simulink model "spacecraft_attitude_model"  (R2024b)
settings: Solver=ode4  StartTime=t0  StopTime=tf  FixedStep=0.1  RelTol=1e-3
values from neighbouring files (symbols this model uses):
  a = (((T/(2*pi))^2*mu_earth)^(1/3))    (= 7069867.85099)    [main_spacecraft_attitude_dynamics.m]
  A_body1 = surface(1)    [main_spacecraft_attitude_dynamics.m]
  A_body2 = surface(2)    [main_spacecraft_attitude_dynamics.m]
  A_body3 = surface(3)    [main_spacecraft_attitude_dynamics.m]
  A_body4 = surface(4)    [main_spacecraft_attitude_dynamics.m]
  A_body5 = surface(5)    [main_spacecraft_attitude_dynamics.m]
  A_body6 = surface(6)    [main_spacecraft_attitude_dynamics.m]
  A_panel1 = surface(7)    [main_spacecraft_attitude_dynamics.m]
  A_panel2 = surface(8)    [main_spacecraft_attitude_dynamics.m]
  A_panel3 = surface(9)    [main_spacecraft_attitude_dynamics.m]
  A_panel4 = surface(10)    [main_spacecraft_attitude_dynamics.m]
  alpha = [alpha1,alpha2,alpha3]    [main_spacecraft_attitude_dynamics.m]
  Ap = pinv(Ar)    [main_spacecraft_attitude_dynamics.m]
  Ar = Ar./norm(Ar)    [main_spacecraft_attitude_dynamics.m]
  AtmosphereModel = struct()    [AtmosphereData.m]    (also in main_spacecraft_attitude_dynamics.m)
  CD = 2.6    [main_spacecraft_attitude_dynamics.m]
  D_max = 50    [main_spacecraft_attitude_dynamics.m]
  Detumbling_time = 5000    [main_spacecraft_attitude_dynamics.m]
  e = 0.001    [main_spacecraft_attitude_dynamics.m]
  FOV = 128 * pi/180    (= 2.23402144255)    [main_spacecraft_attitude_dynamics.m]
  g1_0 = DGRF2020(1).g_nm    [main_spacecraft_attitude_dynamics.m]
  g1_1 = DGRF2020(2).g_nm    [main_spacecraft_attitude_dynamics.m]
  H = 700    [main_spacecraft_attitude_dynamics.m]
  h0 = 0    [main_spacecraft_attitude_dynamics.m]
  h1_1 = DGRF2020(2).h_nm    [main_spacecraft_attitude_dynamics.m]
  i = deg2rad(98.18)    [main_spacecraft_attitude_dynamics.m]
  Ir = 0.1    [main_spacecraft_attitude_dynamics.m]
  J = EXTRACTED_DATA.I_total    [main_spacecraft_attitude_dynamics.m]
  j_B = [0.01, 0.05, 0.01]'    [main_spacecraft_attitude_dynamics.m]
  k1 = max(max(kd_slew))    [main_spacecraft_attitude_dynamics.m]
  k2 = max(max(kp_slew))    [main_spacecraft_attitude_dynamics.m]
  Kw = max(max(kp_detumbling))    [main_spacecraft_attitude_dynamics.m]
  n = sqrt((G*M_E)/(r_earth^3))    [main_spacecraft_attitude_dynamics.m]
  N_B1 = N_B(1, :)'    [main_spacecraft_attitude_dynamics.m]
  N_B2 = N_B(2, :)'    [main_spacecraft_attitude_dynamics.m]
  N_B3 = N_B(3, :)'    [main_spacecraft_attitude_dynamics.m]
  N_B4 = N_B(4, :)'    [main_spacecraft_attitude_dynamics.m]
  N_B5 = N_B(5, :)'    [main_spacecraft_attitude_dynamics.m]
  N_B6 = N_B(6, :)'    [main_spacecraft_attitude_dynamics.m]
  N_P1 = N_B(7, :)'    [main_spacecraft_attitude_dynamics.m]
  N_P2 = N_B(8, :)'    [main_spacecraft_attitude_dynamics.m]
  N_P3 = N_B(9, :)'    [main_spacecraft_attitude_dynamics.m]
  N_P4 = N_B(10, :)'    [main_spacecraft_attitude_dynamics.m]
  n_S = (2*pi)/T_S    (= 1.99238499086e-07)    [main_spacecraft_attitude_dynamics.m]
  om = deg2rad(0)    [main_spacecraft_attitude_dynamics.m]
  P = Fe/c    (= 4.52980041279e-06)    [main_spacecraft_attitude_dynamics.m]
  pd_body1 = rho_D(1)    [main_spacecraft_attitude_dynamics.m]
  pd_body2 = rho_D(2)    [main_spacecraft_attitude_dynamics.m]
  pd_body3 = rho_D(3)    [main_spacecraft_attitude_dynamics.m]
  pd_body4 = rho_D(4)    [main_spacecraft_attitude_dynamics.m]
  pd_body5 = rho_D(5)    [main_spacecraft_attitude_dynamics.m]
  pd_body6 = rho_D(6)    [main_spacecraft_attitude_dynamics.m]
  pd_panel1 = rho_D(7)    [main_spacecraft_attitude_dynamics.m]
  pd_panel2 = rho_D(8)    [main_spacecraft_attitude_dynamics.m]
  pd_panel3 = rho_D(9)    [main_spacecraft_attitude_dynamics.m]
  pd_panel4 = rho_D(10)    [main_spacecraft_attitude_dynamics.m]
  ps_body1 = rho_S(1)    [main_spacecraft_attitude_dynamics.m]
  ps_body2 = rho_S(2)    [main_spacecraft_attitude_dynamics.m]
  ps_body3 = rho_S(3)    [main_spacecraft_attitude_dynamics.m]
  ps_body4 = rho_S(4)    [main_spacecraft_attitude_dynamics.m]
  ps_body5 = rho_S(5)    [main_spacecraft_attitude_dynamics.m]
  ps_body6 = rho_S(6)    [main_spacecraft_attitude_dynamics.m]
  ps_panel1 = rho_S(7)    [main_spacecraft_attitude_dynamics.m]
  ps_panel2 = rho_S(8)    [main_spacecraft_attitude_dynamics.m]
  ps_panel3 = rho_S(9)    [main_spacecraft_attitude_dynamics.m]
  ps_panel4 = rho_S(10)    [main_spacecraft_attitude_dynamics.m]
  q0 = [q1_0 q2_0 q3_0 q4_0]    [main_spacecraft_attitude_dynamics.m]
  r_earth = (R_earth + H)*10^3    (= 7078136.3)    [main_spacecraft_attitude_dynamics.m]
  R_earth = 6378.1363    [main_spacecraft_attitude_dynamics.m]
  r_f1 = r_F(1, :)'    [main_spacecraft_attitude_dynamics.m]
  r_f10 = r_F(10, :)'    [main_spacecraft_attitude_dynamics.m]
  r_f2 = r_F(2, :)'    [main_spacecraft_attitude_dynamics.m]
  r_f3 = r_F(3, :)'    [main_spacecraft_attitude_dynamics.m]
  r_f4 = r_F(4, :)'    [main_spacecraft_attitude_dynamics.m]
  r_f5 = r_F(5, :)'    [main_spacecraft_attitude_dynamics.m]
  r_f6 = r_F(6, :)'    [main_spacecraft_attitude_dynamics.m]
  r_f7 = r_F(7, :)'    [main_spacecraft_attitude_dynamics.m]
  r_f8 = r_F(8, :)'    [main_spacecraft_attitude_dynamics.m]
  r_f9 = r_F(9, :)'    [main_spacecraft_attitude_dynamics.m]
  r_Sun = 149597870    [main_spacecraft_attitude_dynamics.m]
  RAAN = deg2rad(RAAN)    [main_spacecraft_attitude_dynamics.m]
  sigma_b = RRW*(pi/180)*(1/3600)*(1/sqrt(Ts))    [main_spacecraft_attitude_dynamics.m]
  sigma_mag = 10^-6    (= 1e-06)    [main_spacecraft_attitude_dynamics.m]
  sigma_n = ARW*(pi/180)*(1/60)*(1/sqrt(Ts))    [main_spacecraft_attitude_dynamics.m]
  T_coil_max = 50 * 45*10^-6    (= 0.00225)    [main_spacecraft_attitude_dynamics.m]
  th0 = 0    [main_spacecraft_attitude_dynamics.m]
  v0 = [0 0 0]    [main_spacecraft_attitude_dynamics.m]
  variance_Ss = (a_sun)^2    (= 3.24)    [main_spacecraft_attitude_dynamics.m]
  w_0 = [-3, 3, 3]'    [main_spacecraft_attitude_dynamics.m]
  w_E = (2*pi)/(24*60*60)    (= 7.27220521664e-05)    [main_spacecraft_attitude_dynamics.m]
  w_LN = [0 0 0]'    [main_spacecraft_attitude_dynamics.m]
undefined symbols (not defined in the file or in its folder): A_Ss_orienation
libraries: matrix_library x38, slpidlib x2, aerolibutil x1, vrlib x1
(part 1 of 4)
settings Model: Creator=pmarzai02  LastModifiedBy=paolo
settings DebuggingCC: AlgebraicLoopMsg=none

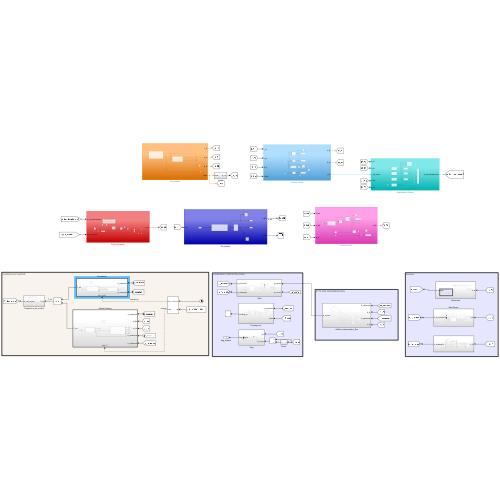
[thumbnail: Simulink's stored preview of the top-level diagram]
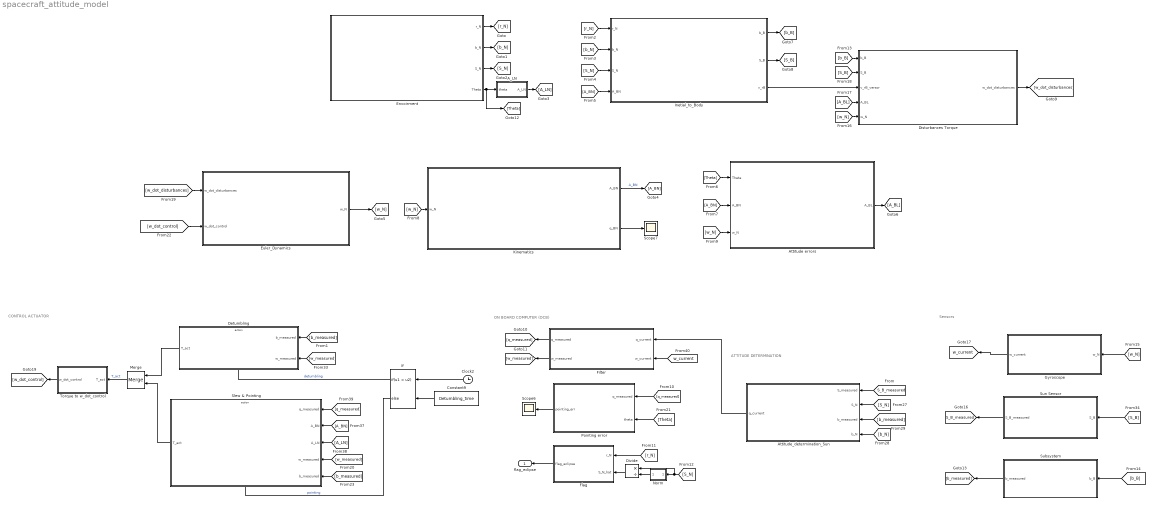
== system spacecraft_attitude_model ==
  note: CONTROL ACTUATOR
  note: ON BOARD COMPUTER (OCB)
  note: Sensors
  note: ATTITUDE DETERMINATION
  " Filter" : Subsystem
  A_LN : Subsystem
  Attitude errors : Subsystem
  Attitude_determination_Sun : Subsystem
  Clock2 : Clock
  Constant9 : Constant  Value=Detumbling_time
  Detumbling : Subsystem  TreatAsAtomicUnit=on
  Disturbances Torque : Subsystem
  Divide : Product  Inputs=*/
  Envoirment : Subsystem
  Euler_Dynamics : Subsystem
  Flag : Subsystem
  Gyroscope : Subsystem
  If : If  NumInputs=2  IfExpression=u1 < u2
  Inetial_to_Body : Subsystem
  Kinematics : Subsystem
  Merge : Merge
  Norm : Subsystem
  Pointing error : Subsystem
  Scope6 : Scope
  Scope7 : Scope
  Slew & Pointing : Subsystem  TreatAsAtomicUnit=on
  Subsystem : Subsystem
  "Sun Sensor " : Subsystem
  Torque to w_dot_control : Subsystem
  flag_eclipse : Outport
  tag scope: S_B_measured=global, w_current=global
  wires:
  Envoirment/1(r_N) -> [r_N]
  Envoirment/2(b_N) -> [b_N]
  Envoirment/3(S_N) -> [S_N]
  [r_N] -> Inetial_to_Body/1(r_N)
  [b_N] -> Inetial_to_Body/2(b_N)
  [S_N] -> Inetial_to_Body/3(S_N)
  Kinematics/1(A_BN) -> [A_BN]  "A_BN"
  [A_BN] -> Inetial_to_Body/4(A_BN)
  [Theta] -> Attitude errors/1(Theta)
  [A_BN] -> Attitude errors/2(A_BN)
  Euler_Dynamics/1(w_N) -> [w_N]
  [w_N] -> Kinematics/1(w_N)
  [w_N] -> Attitude errors/3(w_N)
  [w_N] -> Disturbances Torque/5(w_N)
  [A_BL] -> Disturbances Torque/4(A_BL)
  Attitude errors/1(A_BL) -> [A_BL]
  Inetial_to_Body/1(b_B) -> [b_B]
  Inetial_to_Body/2(S_B) -> [S_B]
  [b_B] -> Disturbances Torque/1(b_B)
  [S_B] -> Disturbances Torque/2(S_B)
  Disturbances Torque/1(w_dot_disturbances) -> [w_dot_disturbances]
  [w_dot_disturbances] -> Euler_Dynamics/1(w_dot_disturbances)
  Subsystem/1(b_measured) -> [b_measured]
  Kinematics/2(q_BN) -> Scope7/1
  Inetial_to_Body/3(v_rB) -> Disturbances Torque/3(v_rB_versor)
  Divide/1 -> Flag/2(S_N_hat)
  [r_N] -> Flag/1(r_N)
  Norm/1(Out1) -> Divide/2
  Flag/1(flag_eclipse) -> flag_eclipse/1
  "Sun Sensor "/1(S_B_measured) -> [S_B_measured]
  [S_B] -> "Sun Sensor "/1(S_B)
  Envoirment/4(Theta) -> [Theta], A_LN/1(theta)
  [b_measured] -> Attitude_determination_Sun/3(b_measured)
  [S_N] -> Attitude_determination_Sun/2(S_N)
  [S_B_measured] -> Attitude_determination_Sun/1(S_measured)
  [b_N] -> Attitude_determination_Sun/4(b_N)
  [w_current] -> " Filter"/2(w_current)
  A_LN/1("A_LN ") -> [A_LN]
  [w_N] -> Gyroscope/1(w_N)
  Gyroscope/1(w_current) -> [w_current]
  [b_B] -> Subsystem/1(b_B)
  [S_N] -> Divide/1, Norm/1(In1)
  " Filter"/1(q_measured) -> [q_measured]
  " Filter"/2(w_measured) -> [w_measured]
  Attitude_determination_Sun/1(q_current) -> " Filter"/1(q_current)
  Constant9/1 -> If/2
  Clock2/1 -> If/1
  If/1 -> Detumbling/Action  "detumbling"
  Detumbling/1(T_act) -> Merge/1
  [b_measured] -> Detumbling/1(b_measured)
  [w_measured] -> Detumbling/2(w_measured)
  [q_measured] -> Pointing error/1(q_measured)
  [Theta] -> Pointing error/2(theta)
  Pointing error/1(pointing_err) -> Scope6/1
  Merge/1 -> Torque to w_dot_control/1(T_act)  "T_act"
  Torque to w_dot_control/1("w_dot_control ") -> [w_dot_control]
  [w_dot_control] -> Euler_Dynamics/2("w_dot_control ")
  If/2 -> Slew & Pointing/Action  "pointing"
  [w_measured] -> Slew & Pointing/4(w_measured)
  [q_measured] -> Slew & Pointing/1(q_measured)
  [A_BN] -> Slew & Pointing/2(A_BN)
  [A_LN] -> Slew & Pointing/3(A_LN)
  [b_measured] -> Slew & Pointing/5(b_measured)
  Slew & Pointing/1(T_act) -> Merge/2

== system spacecraft_attitude_model/ Filter ==
  note: try different Ki and Kp
  q_current : Inport
  w_current : Inport  Port=2
  Clock : Clock
  PID Controller : slpidlib/PID Controller  Controller=PID  Form=Parallel  TimeDomain=Continuous-time  UseExternalTs=off  SampleTime=-1  IntegratorMethod=Forward Euler  FilterMethod=Forward Euler  ControllerParametersSource=internal  P=0.00001  I=0.00000001  UseKiTs=off  D=0  UseExternalDerivativeSource=off  N=100  UseFilter=on  TunerSelectOption=Transfer Function Based (PID Tuner App)  InitialConditionSource=internal  InitialConditionForIntegrator=0  InitialConditionForFilter=0  DifferentiatorICPrevScaledInput=0  ExternalReset=none  TrackingMode=off  Kt=1  LimitOutput=off  SatLimitsSource=internal  UpperSaturationLimit=inf  LowerSaturationLimit=-inf  LinearizeAsGain=on  AntiWindupMode=none  Kb=1  LimitIntegrator=off  UpperIntegratorSaturationLimit=inf  LowerIntegratorSaturationLimit=-inf  POutMin=[]  POutMax=[]  IOutMin=[]  IOutMax=[]  DOutMin=[]  DOutMax=[]  NOutMin=[]  NOutMax=[]  SumOutMin=[]  SumOutMax=[]  SaturationOutMin=[]  SaturationOutMax=[]  PParamMin=[]  PParamMax=[]  IParamMin=[]  IParamMax=[]  DParamMin=[]  DParamMax=[]  NParamMin=[]  NParamMax=[]  KbParamMin=[]  KbParamMax=[]  KtParamMin=[]  KtParamMax=[]  KbOutMin=[]  KbOutMax=[]  KtOutMin=[]  KtOutMax=[]  IntegratorOutMin=[]  IntegratorOutMax=[]  FilterOutMin=[]  FilterOutMax=[]  SumI1OutMin=[]  SumI1OutMax=[]  SumI2OutMin=[]  SumI2OutMax=[]  SumI3OutMin=[]  SumI3OutMax=[]  SumI4OutMin=[]  SumI4OutMax=[]  SumDOutMin=[]  SumDOutMax=[]  DifferentiatorOutMin=[]  DifferentiatorOutMax=[]  FilterDiffOutCoefMin=[]  FilterDiffOutCoefMax=[]  ReciprocalOutMin=[]  ReciprocalOutMax=[]  SumDenOutMin=[]  SumDenOutMax=[]  SumNumOutMin=[]  SumNumOutMax=[]  DivideOutMin=[]  DivideOutMax=[]  UdiffTsProdOutMin=[]  UdiffTsProdOutMax=[]  NTsProdOutMin=[]  NTsProdOutMax=[]  UintegralTsProdOutMin=[]  UintegralTsProdOutMax=[]  UngainTsProdOutMin=[]  UngainTsProdOutMax=[]  ClampingZeroOutDataTypeStr=Inherit: Inherit via back propagation  ClampingZeroOutMin=[]  ClampingZeroOutMax=[]  FilterDenConstantOutDataTypeStr=Inherit: Inherit via back propagation  FilterDenConstantOutMin=[]  FilterDenConstantOutMax=[]  PCopyOutDataTypeStr=Inherit: Inherit via back propagation  PCopyOutMin=[]  PCopyOutMax=[]  NCopyOutDataTypeStr=Inherit: Inherit via back propagation  NCopyOutMin=[]  NCopyOutMax=[]  IntegratorContinuousStateAttributes=''  IntegratorStateMustResolveToSignalObject=off  IntegratorRTWStateStorageClass=Auto  FilterContinuousStateAttributes=''  FilterStateMustResolveToSignalObject=off  FilterRTWStateStorageClass=Auto  ParallelPVariant=InternalParameters  IdealPVariant=Disabled  IVariant=InternalParameters  DVariant=InternalParameters  IntegratorVariant=Continuous  SatVariant=Disabled  AWVariant=Passthrough  PCopyVariant=Disabled  TRVariant=Disabled  FdbkBlocksVariant=Forward  IdealPFdbkVariant=Disabled  SatFdbkVariant=Disabled  DerivativeFilterVariant=ContFilter  NVariant=InternalParameters  NCopyVariant=Disabled  FilterICVariant=InternalICsFilter  IntegratorICVariant=InternalICs  ExternalResetVariant=Disabled  TRSumVariant=Passthrough  SumFdbkVariant=Disabled  SumVariant=Sum_PID  TsampFilterVariant=InternalTs  TsampNgainVariant=Passthrough  TsampIntegralVariant=Disabled_SignalSpec  ExternalSaturationOutDataTypeStr=Inherit: Same as second input  DerivativeSourceVariant=ErrorSignal  PreIntVariant=InternalPreInt
  Quaternions : Subsystem
  Scope : Scope
  Scope2 : Scope
  Scope5 : Scope
  Selector : Selector  InputPortWidth=4  IndexOptions=Index vector (dialog)  Indices=[1:3]  OutputSizes=1
  Subsystem : Subsystem
  Sum : Sum  Inputs=++|
  Switch : Switch  Criteria=u2 > Threshold  SaturateOnIntegerOverflow=off  InputSameDT=off
  To Workspace : ToWorkspace  VariableName=q_measured  SampleTime=-1
  To Workspace1 : ToWorkspace  VariableName=w_measured  SampleTime=-1
  Zero-Order Hold1 : ZeroOrderHold  SampleTime=0.1
  q_measured : Outport
  w_measured : Outport  Port=2
  wires:
  Subsystem/1(q_error) -> Selector/1
  PID Controller/1 -> Scope5/1, Sum/2
  w_current/1 -> Sum/1
  Selector/1 -> PID Controller/1
  Clock/1 -> Switch/2
  Quaternions/1(quaternions) -> Switch/1, Zero-Order Hold1/1
  Switch/1 -> Subsystem/2(q_measured)
  q_current/1 -> Switch/3, Subsystem/1(q_referance)
  Sum/1 -> Quaternions/1(w_current), To Workspace1/1, Scope/1, w_measured/1
  Zero-Order Hold1/1 -> Scope2/1, To Workspace/1, q_measured/1

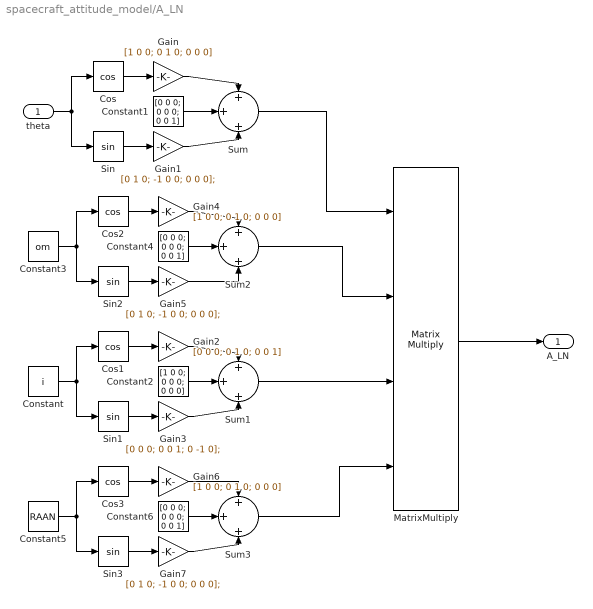
== system spacecraft_attitude_model/A_LN ==
  theta : Inport
  Constant : Constant  Value=i
  Constant1 : Constant  Value=[0 0 0; 0 0 0; 0 0 1]
  Constant2 : Constant  Value=[1 0 0; 0 0 0; 0 0 0]
  Constant3 : Constant  Value=om
  Constant4 : Constant  Value=[0 0 0; 0 0 0; 0 0 1]
  Constant5 : Constant  Value=RAAN
  Constant6 : Constant  Value=[0 0 0; 0 0 0; 0 0 1]
  Cos{,1..3} (4 alike) : Trigonometry  Operator=cos
  Gain : Gain  Gain=[1 0 0; 0 1 0; 0 0 0]
  Gain1 : Gain  Gain=[0 1 0; -1 0 0; 0 0 0];
  Gain2 : Gain  Gain=[0 0 0; 0 1 0; 0 0 1]
  Gain3 : Gain  Gain=[0 0 0; 0 0 1; 0 -1 0];
  Gain4 : Gain  Gain=[1 0 0; 0 1 0; 0 0 0]
  Gain5 : Gain  Gain=[0 1 0; -1 0 0; 0 0 0];
  Gain6 : Gain  Gain=[1 0 0; 0 1 0; 0 0 0]
  Gain7 : Gain  Gain=[0 1 0; -1 0 0; 0 0 0];
  MatrixMultiply : Product  Inputs=4  Multiplication=Matrix(*)
  Sin{,1..3} (4 alike) : Trigonometry
  Sum{,1..3} (4 alike) : Sum  Inputs=+||+||+
  "A_LN " : Outport
  wires:
  theta/1 -> Sin/1, Cos/1
  Cos/1 -> Gain/1
  Sin/1 -> Gain1/1
  Gain1/1 -> Sum/3
  Gain/1 -> Sum/1
  Constant1/1 -> Sum/2
  Sum/1 -> MatrixMultiply/1
  Constant/1 -> Sin1/1, Cos1/1
  Constant2/1 -> Sum1/2
  Sin1/1 -> Gain3/1
  Gain3/1 -> Sum1/3
  Cos1/1 -> Gain2/1
  Sum1/1 -> MatrixMultiply/3
  Gain2/1 -> Sum1/1
  MatrixMultiply/1 -> "A_LN "/1
  Sum2/1 -> MatrixMultiply/2
  Gain4/1 -> Sum2/1
  Cos2/1 -> Gain4/1
  Constant3/1 -> Sin2/1, Cos2/1
  Constant4/1 -> Sum2/2
  Gain5/1 -> Sum2/3
  Sin2/1 -> Gain5/1
  Sum3/1 -> MatrixMultiply/4
  Gain6/1 -> Sum3/1
  Cos3/1 -> Gain6/1
  Constant5/1 -> Sin3/1, Cos3/1
  Constant6/1 -> Sum3/2
  Gain7/1 -> Sum3/3
  Sin3/1 -> Gain7/1

== system spacecraft_attitude_model/Attitude errors ==
  Theta : Inport
  A_BN : Inport  Port=2
  w_N : Inport  Port=3
  A_LN : Subsystem
  Constant : Constant  Value=w_LN
  Gain : Gain  Gain=-1
  Matrix Multiply : Product  Multiplication=Matrix(*)
  Matrix Multiply1 : Product  Multiplication=Matrix(*)
  Scope : Scope
  Scope1 : Scope
  Sum : Sum  Inputs=|++
  To Workspace : ToWorkspace  VariableName=A_BL  SampleTime=-1
  To Workspace1 : ToWorkspace  VariableName=w_BL  SampleTime=-1
  Transpose : matrix_library/Transpose
  A_BL : Outport
  wires:
  A_BN/1 -> Matrix Multiply/1
  Matrix Multiply/1 -> Matrix Multiply1/1, A_BL/1, To Workspace/1, Scope1/1
  Matrix Multiply1/1 -> Gain/1
  Gain/1 -> Sum/2
  w_N/1 -> Sum/1
  Sum/1 -> Scope/1, To Workspace1/1
  A_LN/1(A_LN) -> Transpose/1
  Transpose/1 -> Matrix Multiply/2
  Constant/1 -> Matrix Multiply1/2
  Theta/1 -> A_LN/1(Theta)

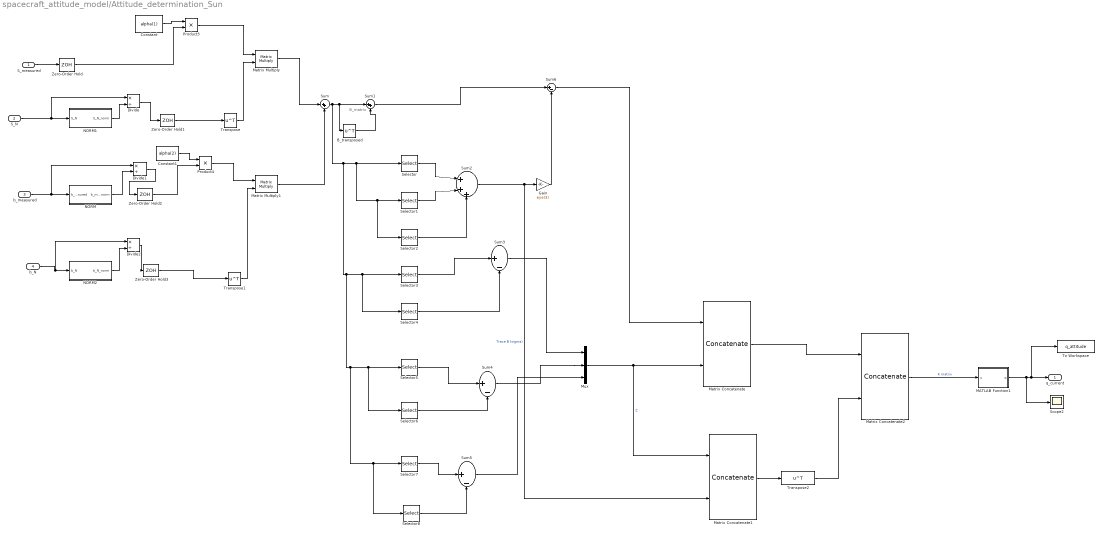
== system spacecraft_attitude_model/Attitude_determination_Sun ==
  note: B_matrix
  S_measured : Inport
  S_N : Inport  Port=2
  b_measured : Inport  Port=3
  b_N : Inport  Port=4
  B_transposed : Math  Operator=transpose
  Constant : Constant  Value=alpha(1)
  Constant1 : Constant  Value=alpha(2)
  Divide : Product  Inputs=*/
  Divide1 : Product  Inputs=*/
  Divide2 : Product  Inputs=*/
  Gain : Gain  Gain=eye(3)
  MATLAB Function1 : MATLAB Function  TreatAsAtomicUnit=on
  Matrix Concatenate : Concatenate  Mode=Multidimensional array  ConcatenateDimension=2
  Matrix Concatenate1 : Concatenate  Mode=Multidimensional array
  Matrix Concatenate2 : Concatenate  Mode=Multidimensional array
  Matrix Multiply : Product  Multiplication=Matrix(*)
  Matrix Multiply1 : Product  Multiplication=Matrix(*)
  Mux : Mux  Inputs=3
  NORM : Subsystem
  NORM1 : Subsystem
  NORM2 : Subsystem
  Product3 : Product
  Product4 : Product
  Scope2 : Scope
  Selector : Selector  NumberOfDimensions=2  InputPortWidth=3  IndexOptions=Index vector (dialog),Index vector (dialog)  Indices=[1],1  OutputSizes=1,1
  Selector1 : Selector  NumberOfDimensions=2  InputPortWidth=3  IndexOptions=Index vector (dialog),Index vector (dialog)  Indices=[2],2  OutputSizes=1,1
  Selector2 : Selector  NumberOfDimensions=2  InputPortWidth=3  IndexOptions=Index vector (dialog),Index vector (dialog)  Indices=[3],3  OutputSizes=1,1
  Selector3 : Selector  NumberOfDimensions=2  InputPortWidth=3  IndexOptions=Index vector (dialog),Index vector (dialog)  Indices=[2],3  OutputSizes=1,1
  Selector4 : Selector  NumberOfDimensions=2  InputPortWidth=3  IndexOptions=Index vector (dialog),Index vector (dialog)  Indices=[3],2  OutputSizes=1,1
  Selector5 : Selector  NumberOfDimensions=2  InputPortWidth=3  IndexOptions=Index vector (dialog),Index vector (dialog)  Indices=[3],1  OutputSizes=1,1
  Selector6 : Selector  NumberOfDimensions=2  InputPortWidth=3  IndexOptions=Index vector (dialog),Index vector (dialog)  Indices=[1],3  OutputSizes=1,1
  Selector7 : Selector  NumberOfDimensions=2  InputPortWidth=3  IndexOptions=Index vector (dialog),Index vector (dialog)  Indices=[1],2  OutputSizes=1,1
  Selector8 : Selector  NumberOfDimensions=2  InputPortWidth=3  IndexOptions=Index vector (dialog),Index vector (dialog)  Indices=[2],1  OutputSizes=1,1
  Sum : Sum  Inputs=|++
  Sum1 : Sum  Inputs=|++
  Sum2 : Sum  Inputs=|+++
  Sum{3..6} (4 alike) : Sum  Inputs=|+-
  To Workspace : ToWorkspace  VariableName=q_attitude  SampleTime=-1
  Transpose : Math  Operator=transpose
  Transpose1 : Math  Operator=transpose
  Transpose2 : Math  Operator=transpose
  Zero-Order Hold{,1..3} (4 alike) : ZeroOrderHold  SampleTime=-1
  q_current : Outport
  wires:
  b_measured/1 -> Divide1/1, NORM/1(b_measured)
  S_N/1 -> Divide/1, NORM1/1(S_N)
  b_N/1 -> Divide2/1, NORM2/1(b_N)
  S_measured/1 -> Zero-Order Hold/1
  Zero-Order Hold/1 -> Product3/2
  Zero-Order Hold1/1 -> Transpose/1
  Zero-Order Hold2/1 -> Product4/2
  Zero-Order Hold3/1 -> Transpose1/1
  NORM1/1(S_N_norm) -> Divide/2
  Divide/1 -> Zero-Order Hold1/1
  NORM/1(b_measured_norm) -> Divide1/2
  Divide1/1 -> Zero-Order Hold2/1
  NORM2/1(b_N_norm) -> Divide2/2
  Divide2/1 -> Zero-Order Hold3/1
  Constant/1 -> Product3/1
  Transpose/1 -> Matrix Multiply/2
  Product3/1 -> Matrix Multiply/1
  Matrix Multiply/1 -> Sum/1
  Constant1/1 -> Product4/1
  Product4/1 -> Matrix Multiply1/1
  Transpose1/1 -> Matrix Multiply1/2
  Matrix Multiply1/1 -> Sum/2
  Sum/1 -> Selector8/1, Selector7/1, Selector6/1, Selector5/1, Selector4/1, Selector3/1, Selector2/1, Selector1/1, Selector/1, Sum1/1, B_transposed/1
  B_transposed/1 -> Sum1/2
  Selector/1 -> Sum2/1
  Selector1/1 -> Sum2/2
  Selector2/1 -> Sum2/3
  Sum2/1 -> Matrix Concatenate1/2, Gain/1  "Trace B (sigma)"
  Selector3/1 -> Sum3/1
  Selector4/1 -> Sum3/2
  Selector5/1 -> Sum4/1
  Selector6/1 -> Sum4/2
  Selector7/1 -> Sum5/1
  Selector8/1 -> Sum5/2
  Sum3/1 -> Mux/1
  Sum4/1 -> Mux/2
  Sum5/1 -> Mux/3
  Mux/1 -> Matrix Concatenate1/1, Matrix Concatenate/2  "Z"
  Sum1/1 -> Sum6/1
  Gain/1 -> Sum6/2
  Sum6/1 -> Matrix Concatenate/1
  Matrix Concatenate1/1 -> Transpose2/1
  Matrix Concatenate/1 -> Matrix Concatenate2/1
  Transpose2/1 -> Matrix Concatenate2/2
  Matrix Concatenate2/1 -> MATLAB Function1/1(u)  "K matrix"
  MATLAB Function1/1(q) -> Scope2/1, To Workspace/1, q_current/1

== system spacecraft_attitude_model/Detumbling ==
  b_measured : Inport
  w_measured : Inport  Port=2
  Action Port : ActionPort  ActionPortLabel=if(u1 < u2)
  Detumbling : Subsystem
  Subsystem4 : Subsystem
  T_act : Outport
  wires:
  b_measured/1 -> Subsystem4/2(b_measured)
  Detumbling/1(T_detumbling) -> Subsystem4/1(T_control)
  w_measured/1 -> Subsystem4/3(w_measured), Detumbling/1(w_measured)
  Subsystem4/1(T_act) -> T_act/1

== system spacecraft_attitude_model/Disturbances Torque ==
  b_B : Inport
  S_B : Inport  Port=2
  v_rB_versor : Inport  Port=3
  A_BL : Inport  Port=4
  w_N : Inport  Port=5
  Air Drag : Subsystem
  Gain{,1..3} (4 alike) : Gain
  Gravity Gradient : Subsystem
  Magnetic_Torque : Subsystem
  Scope : Scope  NumInputPorts=4
  Solar_Radiation_Torque : Subsystem
  Sum : Sum  Inputs=|++++
  torque to w_dot_B : Subsystem
  torque to w_dot_Drag : Subsystem
  torque to w_dot_SRP : Subsystem
  w_dot_disturbances : Outport
  wires:
  Solar_Radiation_Torque/1(T sun) -> Scope/2, torque to w_dot_SRP/1(T_S)  "T_SRP"
  Gravity Gradient/1(w_dot_GG) -> Gain3/1
  Gain1/1 -> Sum/2
  w_N/1 -> Gravity Gradient/2(w)
  b_B/1 -> Magnetic_Torque/1(b_B)
  Gain2/1 -> Sum/3
  Gain3/1 -> Sum/4
  Air Drag/1(T_Drag) -> Scope/3, torque to w_dot_Drag/1(T_Drag)  "T_DRAG"
  torque to w_dot_SRP/1("w_dot_SRP ") -> Gain/1
  torque to w_dot_B/1(w_dot_B) -> Gain1/1
  Gain/1 -> Sum/1
  torque to w_dot_Drag/1(w_dot_Drag) -> Gain2/1
  v_rB_versor/1 -> Air Drag/1(v_rB_versor)
  A_BL/1 -> Gravity Gradient/1(A_BL)
  S_B/1 -> Solar_Radiation_Torque/1(S_B)
  Sum/1 -> w_dot_disturbances/1
  Gravity Gradient/2("T_GG ") -> Scope/4  "T_GG"
  Magnetic_Torque/1(T_B) -> Scope/1, torque to w_dot_B/1(T_B)  "T_M"

== system spacecraft_attitude_model/Envoirment ==
  Model : Subsystem
  Scope : Scope
  Two_Body_Keplerian_Dynamics : Subsystem
  r_N : Outport
  b_N : Outport  Port=2
  S_N : Outport  Port=3
  Theta : Outport  Port=4
  wires:
  Two_Body_Keplerian_Dynamics/1(r_N) -> r_N/1, Model/1(r_N)
  Model/1(b_N) -> Scope/1, b_N/1
  Model/2(S_N) -> S_N/1
  Two_Body_Keplerian_Dynamics/2(Theta) -> Theta/1

== system spacecraft_attitude_model/Euler_Dynamics ==
  note: Euler's equation in vectorial forme
      | $I*\underline{\dot{\omega}} + \underline{{\omega}} \times (I * \underline{{\omega}}) = T$
      | It has needed a vector of initial angular speed $\omega_0$
      | $\underline{\dot{\omega}} = I^{-1}*[T-(\underline{{\omega}}\times I)*\underline{{\omega}}]$
  w_dot_disturbances : Inport
  "w_dot_control " : Inport  Port=2
  Constant : Constant  Value=J
  Constant1 : Constant  Value=inv(J)
  Cross Product : matrix_library/Cross Product
  Gain : Gain  Gain=+1
  Integrator : Integrator  InitialCondition=w_0
  Product3 : Product  Multiplication=Matrix(*)
  Product4 : Product  Multiplication=Matrix(*)
  Scope : Scope
  Sum1 : Sum  Inputs=|+++
  To Workspace1 : ToWorkspace  VariableName=w  SampleTime=-1
  Transpose : Math  Operator=transpose
  Transpose1 : Math  Operator=transpose
  w_N : Outport
  wires:
  Cross Product/1 -> Product4/2
  Constant1/1 -> Product4/1
  Constant/1 -> Product3/1
  Product3/1 -> Cross Product/1
  Integrator/1 -> Scope/1, Cross Product/2, Product3/2, To Workspace1/1, w_N/1  "w"
  Product4/1 -> Sum1/1
  Sum1/1 -> Integrator/1
  w_dot_disturbances/1 -> Transpose/1  "w_dot_distrubance"
  Transpose/1 -> Sum1/2
  "w_dot_control "/1 -> Gain/1
  Transpose1/1 -> Sum1/3
  Gain/1 -> Transpose1/1  "w_dot_control"

== system spacecraft_attitude_model/Flag ==
  note: Here we are checking the angle between r_N and S_N and also if the distance between directions is smaller than the earth radius
  r_N : Inport
  S_N_hat : Inport  Port=2
  Constant1 : Constant  Value=0
  Constant2 : Constant
  Dot Product : DotProduct  OutDataTypeStr=Inherit: Inherit via internal rule
  Dot Product1 : DotProduct  OutDataTypeStr=Inherit: Inherit via internal rule
  Dot Product2 : DotProduct  OutDataTypeStr=Inherit: Inherit via internal rule
  Product1 : Product
  Product2 : Product
  Square Root : Sqrt
  Square Root1 : Sqrt
  Sum1 : Sum  Inputs=|+-
  Switch : Switch  Criteria=u2 > Threshold  SaturateOnIntegerOverflow=off  InputSameDT=off
  Switch1 : Switch  Criteria=u2 > Threshold  Threshold=R_earth  SaturateOnIntegerOverflow=off  InputSameDT=off
  flag_eclipse : Outport
  wires:
  Product1/1 -> Switch/2
  Dot Product/1 -> Square Root/1
  Product2/1 -> Sum1/2
  Sum1/1 -> Dot Product2/1, Dot Product2/2
  r_N/1 -> Sum1/1, Dot Product1/1, Dot Product/2, Dot Product/1
  Constant1/1 -> Switch1/1, Switch/1
  S_N_hat/1 -> Product1/2, Dot Product1/2, Product2/2
  Square Root/1 -> Product1/1
  Constant2/1 -> Switch/3
  Square Root1/1 -> Switch1/2
  Dot Product2/1 -> Square Root1/1
  Switch/1 -> Switch1/3
  Switch1/1 -> flag_eclipse/1
  Dot Product1/1 -> Product2/1

== system spacecraft_attitude_model/Gyroscope ==
  note: Noise
  w_N : Inport
  Add : Sum
  Add1 : Sum
  Integrator : Integrator
  Saturation : Saturate  UpperLimit=400*pi/180  LowerLimit=-400*pi/180
  Scope1 : Scope
  Zero-Order Hold : ZeroOrderHold  SampleTime=0.1
  b : RandomNumber  Variance=sigma_b^2  SampleTime=0.1
  n : RandomNumber  Variance=sigma_n^2  SampleTime=0.1
  w_current : Outport
  wires:
  w_N/1 -> Add/1
  Integrator/1 -> Add1/2
  n/1 -> Add1/1
  b/1 -> Integrator/1
  Add1/1 -> Add/2
  Add/1 -> Saturation/1
  Saturation/1 -> Zero-Order Hold/1
  Zero-Order Hold/1 -> w_current/1, Scope1/1

== system spacecraft_attitude_model/Inetial_to_Body ==
  r_N : Inport
  b_N : Inport  Port=2
  S_N : Inport  Port=3
  A_BN : Inport  Port=4
  Matrix Multiply{,1..3} (4 alike) : Product  Multiplication=Matrix(*)
  Scope : Scope
  Scope1 : Scope
  To Workspace : ToWorkspace  VariableName=b_B  SampleTime=-1
  To Workspace1 : ToWorkspace  VariableName=r_B  SampleTime=-1
  To Workspace2 : ToWorkspace  VariableName=S_B  SampleTime=-1
  Transpose1 : Math  Operator=transpose
  v_rel : Subsystem
  b_B : Outport
  S_B : Outport  Port=2
  v_rB : Outport  Port=3
  wires:
  b_N/1 -> Matrix Multiply/2
  A_BN/1 -> Matrix Multiply/1, Matrix Multiply1/1, Matrix Multiply3/1, Matrix Multiply2/1
  Matrix Multiply/1 -> To Workspace/1, b_B/1, Scope/1
  r_N/1 -> v_rel/1(r_N), Matrix Multiply1/2
  Matrix Multiply1/1 -> To Workspace1/1
  Matrix Multiply2/1 -> S_B/1, Scope1/1, To Workspace2/1
  S_N/1 -> Matrix Multiply2/2
  Transpose1/1 -> Matrix Multiply3/2
  Matrix Multiply3/1 -> v_rB/1
  v_rel/1(v_rN) -> Transpose1/1

== system spacecraft_attitude_model/Kinematics ==
  w_N : Inport
  Scope : Scope
  Scope1 : Scope
  quaternions : Subsystem
  quaternions to DCM : Subsystem
  A_BN : Outport
  q_BN : Outport  Port=2
  wires:
  w_N/1 -> quaternions/1(w)
  quaternions/1(q) -> Scope1/1, q_BN/1, quaternions to DCM/1(q)
  quaternions to DCM/1(A_BN) -> Scope/1, A_BN/1

== system spacecraft_attitude_model/Norm ==
  In1 : Inport
  Demux : Demux  Outputs=3
  Sqrt : Sqrt
  Square : Math  Operator=square
  Square1 : Math  Operator=square
  Square2 : Math  Operator=square
  Sum : Sum  Inputs=|+++
  Out1 : Outport
  wires:
  Demux/3 -> Square2/1
  In1/1 -> Demux/1
  Demux/1 -> Square/1
  Demux/2 -> Square1/1
  Square/1 -> Sum/1
  Square1/1 -> Sum/2
  Square2/1 -> Sum/3
  Sum/1 -> Sqrt/1
  Sqrt/1 -> Out1/1

== system spacecraft_attitude_model/Pointing error ==
  q_measured : Inport
  theta : Inport  Port=2
  A_BL : Scope
  DCM err (1) : Subsystem
  Subsystem1 : Subsystem
  Subsystem2 : Subsystem
  To Workspace : ToWorkspace  VariableName=pointingerror  SampleTime=-1
  To Workspace3 : ToWorkspace  VariableName=q_BL  SampleTime=-1
  q_BL : Scope
  q_LN1 : Subsystem
  pointing_err : Outport
  wires:
  q_measured/1 -> Subsystem1/1(q_BN_sensed)
  DCM err (1)/1(err) -> pointing_err/1, To Workspace/1  "Pnt_err"
  q_LN1/1(q_LN) -> Subsystem1/2(q_LN)
  Subsystem2/1(A_BL) -> A_BL/1, DCM err (1)/1(A_ref)
  Subsystem1/1(q_BL) -> To Workspace3/1, Subsystem2/1(q_BL), q_BL/1  "q_BL"
  theta/1 -> q_LN1/1(theta)

== system spacecraft_attitude_model/Slew & Pointing ==
  q_measured : Inport
  A_BN : Inport  Port=2
  A_LN : Inport  Port=3
  w_measured : Inport  Port=4
  b_measured : Inport  Port=5
  Action Port : ActionPort  ActionPortLabel=else
  Slew and Pointing : Subsystem
  Subsystem : Subsystem
  T_act : Outport
  wires:
  w_measured/1 -> Subsystem/3(w_measured), Slew and Pointing/4(w_measured)
  Slew and Pointing/1(T_c) -> Subsystem/2(T_control)
  A_LN/1 -> Slew and Pointing/3(A_LN)
  q_measured/1 -> Slew and Pointing/1(q_measured)
  A_BN/1 -> Slew and Pointing/2(A_BN)
  b_measured/1 -> Subsystem/1(b_measured)
  Subsystem/1(T_act) -> T_act/1

== system spacecraft_attitude_model/Subsystem ==
  b_B : Inport
  Demux : Demux  Outputs=3
  Mux : Mux  Inputs=3
  Quantizer1 : Quantizer  QuantizationInterval=(1600/2^16)*10^-6
  Random Number1 : RandomNumber  Variance=sigma_mag^2  SampleTime=0.1
  Random Number2 : RandomNumber  Variance=sigma_mag^2  SampleTime=0.1
  Random Number4 : RandomNumber  Variance=sigma_mag^2  SampleTime=0.1
  Sum : Sum  Inputs=|++
  Sum1 : Sum  Inputs=|++
  Sum2 : Sum  Inputs=|++
  To Workspace : ToWorkspace  VariableName=b_measured  SampleTime=-1
  Zero-Order Hold : ZeroOrderHold  SampleTime=0.1
  b_measured : Outport
  wires:
  Quantizer1/1 -> To Workspace/1, b_measured/1
  Random Number1/1 -> Sum1/1
  Random Number4/1 -> Sum/1
  Demux/2 -> Sum1/2
  Sum2/1 -> Mux/3
  Zero-Order Hold/1 -> Demux/1
  Demux/3 -> Sum2/2
  Sum1/1 -> Mux/2
  Demux/1 -> Sum/2
  Random Number2/1 -> Sum2/1
  Sum/1 -> Mux/1
  Mux/1 -> Quantizer1/1
  b_B/1 -> Zero-Order Hold/1

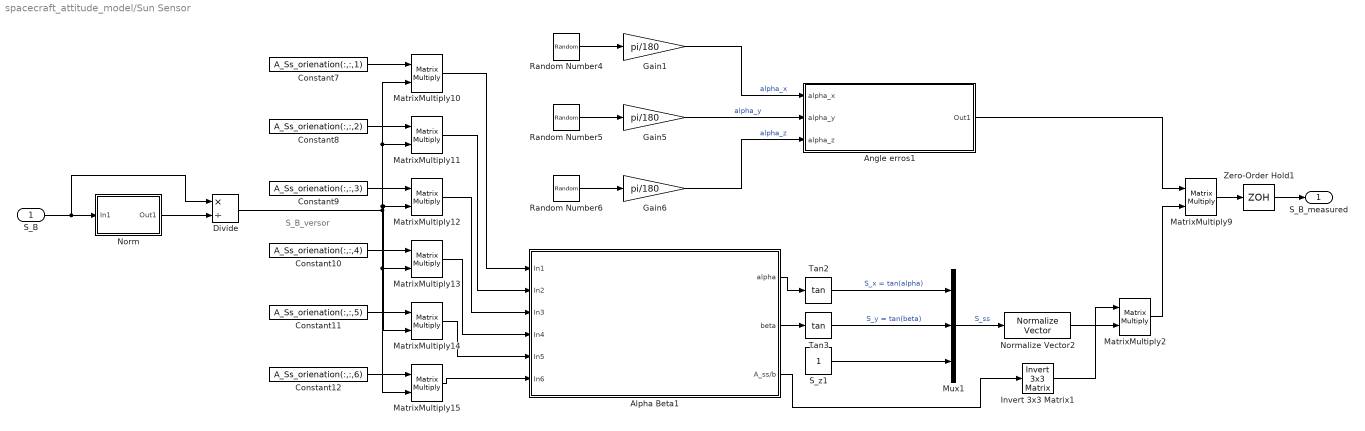
== system spacecraft_attitude_model/Sun Sensor  ==
  note: S_B_versor
  S_B : Inport
  Alpha Beta1 : Subsystem
  Angle erros1 : Subsystem
  Constant10 : Constant  Value=A_Ss_orienation(:,:,4)
  Constant11 : Constant  Value=A_Ss_orienation(:,:,5)
  Constant12 : Constant  Value=A_Ss_orienation(:,:,6)
  Constant7 : Constant  Value=A_Ss_orienation(:,:,1)  VectorParams1D=off
  Constant8 : Constant  Value=A_Ss_orienation(:,:,2)
  Constant9 : Constant  Value=A_Ss_orienation(:,:,3)
  Divide : Product  Inputs=*/
  Gain1 : Gain  Gain=pi/180
  Gain5 : Gain  Gain=pi/180
  Gain6 : Gain  Gain=pi/180
  Invert 3x3 Matrix1 : aerolibutil/Invert  3x3 Matrix
  MatrixMultiply{2,9..15} (8 alike) : Product  Multiplication=Matrix(*)
  Mux1 : Mux  Inputs=3
  Norm : Subsystem
  Normalize Vector2 : vrlib/Utilities/Normalize Vector  maxzero=0
  Random Number4 : RandomNumber  Variance=variance_Ss  SampleTime=0.1
  Random Number5 : RandomNumber  Variance=variance_Ss  SampleTime=0.1
  Random Number6 : RandomNumber  Variance=variance_Ss  SampleTime=0.1
  S_z1 : Constant
  Tan2 : Trigonometry  Operator=tan
  Tan3 : Trigonometry  Operator=tan
  Zero-Order Hold1 : ZeroOrderHold  SampleTime=0.1
  S_B_measured : Outport
  wires:
  Random Number4/1 -> Gain1/1
  S_B/1 -> Norm/1(In1), Divide/1
  MatrixMultiply14/1 -> Alpha Beta1/5(In5)
  Gain6/1 -> Angle erros1/3(alpha_z)  "alpha_z"
  Constant7/1 -> MatrixMultiply10/1
  Mux1/1 -> Normalize Vector2/1  "S_ss"
  Angle erros1/1(Out1) -> MatrixMultiply9/1
  MatrixMultiply10/1 -> Alpha Beta1/1(In1)
  MatrixMultiply11/1 -> Alpha Beta1/2(In2)
  Alpha Beta1/2(beta) -> Tan3/1
  Constant12/1 -> MatrixMultiply15/1
  MatrixMultiply13/1 -> Alpha Beta1/4(In4)
  Constant11/1 -> MatrixMultiply14/1
  Invert 3x3 Matrix1/1 -> MatrixMultiply2/1
  Tan2/1 -> Mux1/1  "S_x = tan(alpha)"
  MatrixMultiply15/1 -> Alpha Beta1/6(In6)
  Gain5/1 -> Angle erros1/2(alpha_y)  "alpha_y"
  MatrixMultiply2/1 -> MatrixMultiply9/2
  Gain1/1 -> Angle erros1/1(alpha_x)  "alpha_x"
  Constant9/1 -> MatrixMultiply12/1
  Zero-Order Hold1/1 -> S_B_measured/1
  Tan3/1 -> Mux1/2  "S_y = tan(beta)"
  MatrixMultiply12/1 -> Alpha Beta1/3(In3)
  Normalize Vector2/1 -> MatrixMultiply2/2
  Alpha Beta1/1(alpha) -> Tan2/1
  Random Number6/1 -> Gain6/1
  MatrixMultiply9/1 -> Zero-Order Hold1/1
  Constant10/1 -> MatrixMultiply13/1
  Random Number5/1 -> Gain5/1
  Alpha Beta1/3(A_ss/b) -> Invert 3x3 Matrix1/1
  S_z1/1 -> Mux1/3
  Constant8/1 -> MatrixMultiply11/1
  Divide/1 -> MatrixMultiply11/2, MatrixMultiply10/2, MatrixMultiply14/2, MatrixMultiply12/2, MatrixMultiply15/2, MatrixMultiply13/2
  Norm/1(Out1) -> Divide/2

== system spacecraft_attitude_model/Torque to w_dot_control ==
  T_act : Inport
  To Workspace : ToWorkspace  VariableName=T_act  SampleTime=-1
  Torque to w_dot : Subsystem
  Transpose : Math  Operator=transpose
  "w_dot_control " : Outport
  wires:
  Transpose/1 -> Torque to w_dot/1(T_c)
  T_act/1 -> To Workspace/1, Transpose/1
  Torque to w_dot/1("w_dot_control ") -> "w_dot_control "/1

== system spacecraft_attitude_model/ Filter/Quaternions ==
  w_current : Inport
  Demux : Demux  Outputs=3
  Gain : Gain  Gain=[0 0 0 1; 0 0 1 0; 0 -1 0 0; -1 0 0 0]
  Gain1 : Gain  Gain=[0 0 -1 0; 0 0 0 1; 1 0 0 0; 0 -1 0 0]
  Gain2 : Gain  Gain=[0 1 0 0; -1 0 0 0; 0 0 0 1; 0 0 -1 0]
  Gain3 : Gain  Gain=1/2
  Integrator : Integrator  InitialCondition=q0
  MatrixMultiply : Product  Multiplication=Matrix(*)
  Sum : Sum  Inputs=+|+|+
  quaternions : Outport
  wires:
  w_current/1 -> Demux/1
  Demux/1 -> Gain/1
  Demux/2 -> Gain1/1
  Demux/3 -> Gain2/1
  Gain/1 -> Sum/1
  Gain1/1 -> Sum/2
  Gain2/1 -> Sum/3
  Gain3/1 -> Integrator/1
  Integrator/1 -> MatrixMultiply/2, quaternions/1  "q"
  MatrixMultiply/1 -> Gain3/1
  Sum/1 -> MatrixMultiply/1

== system spacecraft_attitude_model/ Filter/Subsystem ==
  q_referance : Inport
  q_measured : Inport  Port=2
  Demux : Demux
  Gain : Gain  Gain=[0 0 0 -1; 0 0 1 0; 0 -1 0 0; 1 0 0 0];
  Gain1 : Gain  Gain=[0 1 0 0; -1 0 0 0; 0 0 0 -1; 0 0 1 0];
  Gain2 : Gain  Gain=[0 0 -1 0; 0 0 0 -1; 1 0 0 0; 0 1 0 0];
  Gain3 : Gain  Gain=[1 0 0 0; 0 1 0 0; 0 0 1 0; 0 0 0 1];
  MatrixMultiply : Product  Multiplication=Matrix(*)
  Sum : Sum  Inputs=++++
  q_error : Outport
  wires:
  q_referance/1 -> Demux/1
  Demux/1 -> Gain/1
  Demux/3 -> Gain1/1
  Demux/2 -> Gain2/1
  Demux/4 -> Gain3/1
  Gain/1 -> Sum/1
  Gain2/1 -> Sum/2
  Gain1/1 -> Sum/3
  Gain3/1 -> Sum/4
  Sum/1 -> MatrixMultiply/1
  q_measured/1 -> MatrixMultiply/2
  MatrixMultiply/1 -> q_error/1

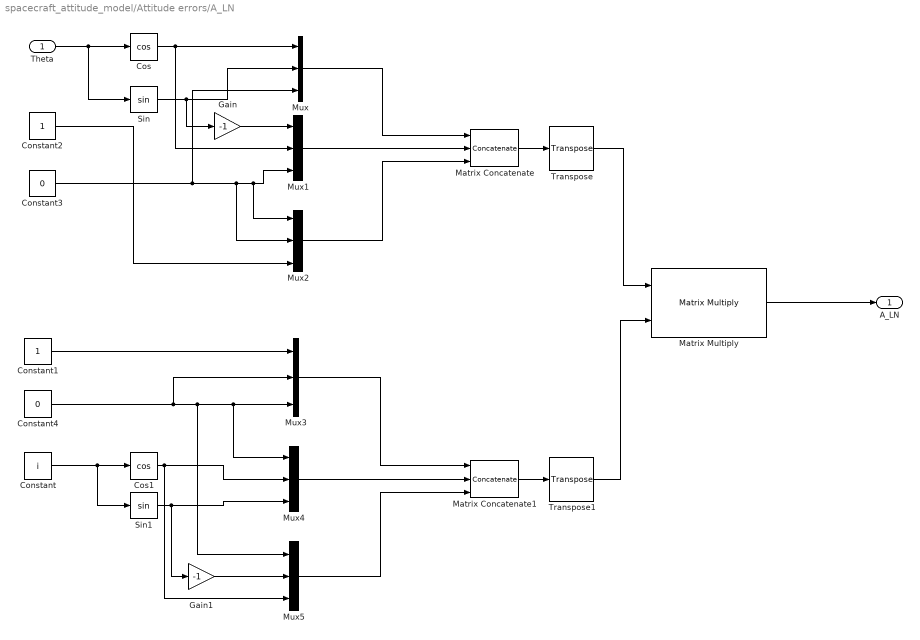
== system spacecraft_attitude_model/Attitude errors/A_LN ==
  Theta : Inport
  Constant : Constant  Value=i
  Constant1 : Constant
  Constant2 : Constant
  Constant3 : Constant  Value=0
  Constant4 : Constant  Value=0
  Cos : Trigonometry  Operator=cos
  Cos1 : Trigonometry  Operator=cos
  Gain : Gain  Gain=-1
  Gain1 : Gain  Gain=-1
  Matrix Concatenate : Concatenate  NumInputs=3  Mode=Multidimensional array  ConcatenateDimension=2
  Matrix Concatenate1 : Concatenate  NumInputs=3  Mode=Multidimensional array  ConcatenateDimension=2
  Matrix Multiply : Product  Multiplication=Matrix(*)
  Mux{,1..5} (6 alike) : Mux  Inputs=3
  Sin : Trigonometry
  Sin1 : Trigonometry
  Transpose : matrix_library/Transpose
  Transpose1 : matrix_library/Transpose
  A_LN : Outport
  wires:
  Theta/1 -> Sin/1, Cos/1
  Constant/1 -> Sin1/1, Cos1/1
  Cos/1 -> Mux/1, Mux1/2
  Sin/1 -> Gain/1, Mux/2
  Constant3/1 -> Mux2/2, Mux2/1, Mux1/3, Mux/3
  Gain/1 -> Mux1/1
  Constant2/1 -> Mux2/3
  Constant1/1 -> Mux3/1
  Constant4/1 -> Mux5/1, Mux4/1, Mux3/3, Mux3/2
  Cos1/1 -> Mux5/3, Mux4/2
  Sin1/1 -> Gain1/1, Mux4/3
  Gain1/1 -> Mux5/2
  Mux/1 -> Matrix Concatenate/1
  Mux1/1 -> Matrix Concatenate/2
  Mux2/1 -> Matrix Concatenate/3
  Mux3/1 -> Matrix Concatenate1/1
  Mux4/1 -> Matrix Concatenate1/2
  Mux5/1 -> Matrix Concatenate1/3
  Matrix Multiply/1 -> A_LN/1
  Matrix Concatenate/1 -> Transpose/1
  Transpose/1 -> Matrix Multiply/1
  Matrix Concatenate1/1 -> Transpose1/1
  Transpose1/1 -> Matrix Multiply/2

== system spacecraft_attitude_model/Attitude_determination_Sun/NORM ==
  b_measured : Inport
  Demux : Demux  Outputs=3
  Sqrt : Sqrt
  Square : Math  Operator=square
  Square1 : Math  Operator=square
  Square2 : Math  Operator=square
  Sum : Sum  Inputs=|+++
  b_measured_norm : Outport
  wires:
  Square1/1 -> Sum/2
  Square2/1 -> Sum/3
  Demux/1 -> Square/1
  Demux/2 -> Square1/1
  Sqrt/1 -> b_measured_norm/1
  Demux/3 -> Square2/1
  Sum/1 -> Sqrt/1
  Square/1 -> Sum/1
  b_measured/1 -> Demux/1

== system spacecraft_attitude_model/Attitude_determination_Sun/NORM1 ==
  S_N : Inport
  Demux : Demux  Outputs=3
  Sqrt : Sqrt
  Square : Math  Operator=square
  Square1 : Math  Operator=square
  Square2 : Math  Operator=square
  Sum : Sum  Inputs=|+++
  S_N_norm : Outport
  wires:
  Square1/1 -> Sum/2
  Square2/1 -> Sum/3
  Demux/1 -> Square/1
  Demux/2 -> Square1/1
  Sqrt/1 -> S_N_norm/1
  Demux/3 -> Square2/1
  Sum/1 -> Sqrt/1
  S_N/1 -> Demux/1
  Square/1 -> Sum/1

== system spacecraft_attitude_model/Attitude_determination_Sun/NORM2 ==
  b_N : Inport
  Demux : Demux  Outputs=3
  Sqrt : Sqrt
  Square : Math  Operator=square
  Square1 : Math  Operator=square
  Square2 : Math  Operator=square
  Sum : Sum  Inputs=|+++
  b_N_norm : Outport
  wires:
  Square1/1 -> Sum/2
  Square2/1 -> Sum/3
  Demux/1 -> Square/1
  Demux/2 -> Square1/1
  Sqrt/1 -> b_N_norm/1
  Demux/3 -> Square2/1
  Sum/1 -> Sqrt/1
  b_N/1 -> Demux/1
  Square/1 -> Sum/1

== system spacecraft_attitude_model/Detumbling/Detumbling ==
  w_measured : Inport
  Gain : Gain  Gain=-1
  PID Controller1 : slpidlib/PID Controller  Controller=PID  Form=Parallel  TimeDomain=Continuous-time  UseExternalTs=off  SampleTime=-1  IntegratorMethod=Forward Euler  FilterMethod=Forward Euler  ControllerParametersSource=internal  P=Kw  I=0  UseKiTs=off  D=0  UseExternalDerivativeSource=off  N=100  UseFilter=on  TunerSelectOption=Transfer Function Based (PID Tuner App)  InitialConditionSource=internal  InitialConditionForIntegrator=0  InitialConditionForFilter=0  DifferentiatorICPrevScaledInput=0  ExternalReset=none  TrackingMode=off  Kt=1  LimitOutput=off  SatLimitsSource=internal  UpperSaturationLimit=inf  LowerSaturationLimit=-inf  LinearizeAsGain=on  AntiWindupMode=none  Kb=1  LimitIntegrator=off  UpperIntegratorSaturationLimit=inf  LowerIntegratorSaturationLimit=-inf  POutMin=[]  POutMax=[]  IOutMin=[]  IOutMax=[]  DOutMin=[]  DOutMax=[]  NOutMin=[]  NOutMax=[]  SumOutMin=[]  SumOutMax=[]  SaturationOutMin=[]  SaturationOutMax=[]  PParamMin=[]  PParamMax=[]  IParamMin=[]  IParamMax=[]  DParamMin=[]  DParamMax=[]  NParamMin=[]  NParamMax=[]  KbParamMin=[]  KbParamMax=[]  KtParamMin=[]  KtParamMax=[]  KbOutMin=[]  KbOutMax=[]  KtOutMin=[]  KtOutMax=[]  IntegratorOutMin=[]  IntegratorOutMax=[]  FilterOutMin=[]  FilterOutMax=[]  SumI1OutMin=[]  SumI1OutMax=[]  SumI2OutMin=[]  SumI2OutMax=[]  SumI3OutMin=[]  SumI3OutMax=[]  SumI4OutMin=[]  SumI4OutMax=[]  SumDOutMin=[]  SumDOutMax=[]  DifferentiatorOutMin=[]  DifferentiatorOutMax=[]  FilterDiffOutCoefMin=[]  FilterDiffOutCoefMax=[]  ReciprocalOutMin=[]  ReciprocalOutMax=[]  SumDenOutMin=[]  SumDenOutMax=[]  SumNumOutMin=[]  SumNumOutMax=[]  DivideOutMin=[]  DivideOutMax=[]  UdiffTsProdOutMin=[]  UdiffTsProdOutMax=[]  NTsProdOutMin=[]  NTsProdOutMax=[]  UintegralTsProdOutMin=[]  UintegralTsProdOutMax=[]  UngainTsProdOutMin=[]  UngainTsProdOutMax=[]  ClampingZeroOutDataTypeStr=Inherit: Inherit via back propagation  ClampingZeroOutMin=[]  ClampingZeroOutMax=[]  FilterDenConstantOutDataTypeStr=Inherit: Inherit via back propagation  FilterDenConstantOutMin=[]  FilterDenConstantOutMax=[]  PCopyOutDataTypeStr=Inherit: Inherit via back propagation  PCopyOutMin=[]  PCopyOutMax=[]  NCopyOutDataTypeStr=Inherit: Inherit via back propagation  NCopyOutMin=[]  NCopyOutMax=[]  IntegratorContinuousStateAttributes=''  IntegratorStateMustResolveToSignalObject=off  IntegratorRTWStateStorageClass=Auto  FilterContinuousStateAttributes=''  FilterStateMustResolveToSignalObject=off  FilterRTWStateStorageClass=Auto  ParallelPVariant=InternalParameters  IdealPVariant=Disabled  IVariant=InternalParameters  DVariant=InternalParameters  IntegratorVariant=Continuous  SatVariant=Disabled  AWVariant=Passthrough  PCopyVariant=Disabled  TRVariant=Disabled  FdbkBlocksVariant=Forward  IdealPFdbkVariant=Disabled  SatFdbkVariant=Disabled  DerivativeFilterVariant=ContFilter  NVariant=InternalParameters  NCopyVariant=Disabled  FilterICVariant=InternalICsFilter  IntegratorICVariant=InternalICs  ExternalResetVariant=Disabled  TRSumVariant=Passthrough  SumFdbkVariant=Disabled  SumVariant=Sum_PID  TsampFilterVariant=InternalTs  TsampNgainVariant=Passthrough  TsampIntegralVariant=Disabled_SignalSpec  ExternalSaturationOutDataTypeStr=Inherit: Same as second input  DerivativeSourceVariant=ErrorSignal  PreIntVariant=InternalPreInt
  Scope : Scope
  T_detumbling : Outport
  wires:
  PID Controller1/1 -> Scope/1, T_detumbling/1  "T_detumbling"
  w_measured/1 -> Gain/1
  Gain/1 -> PID Controller1/1

== system spacecraft_attitude_model/Detumbling/Subsystem4 ==
  T_control : Inport
  b_measured : Inport  Port=2
  w_measured : Inport  Port=3
  Constant : Constant  Value=Ar
  Gain : Gain
  Inertia Wheel : Subsystem
  Magnetic coils : Subsystem
  Product : Product
  Scope : Scope  NumInputPorts=2
  Subtract : Sum  Inputs=+-
  Sum : Sum  Inputs=|++
  To Workspace : ToWorkspace  VariableName=T_wheel_det  SampleTime=-1
  To Workspace1 : ToWorkspace  VariableName=T_coils_det  SampleTime=-1
  T_act : Outport
  wires:
  Sum/1 -> Gain/1
  Gain/1 -> T_act/1
  T_control/1 -> Product/2, Subtract/1
  Inertia Wheel/1(T_wheel) -> To Workspace/1, Sum/1
  Product/1 -> Subtract/2, Scope/1, Inertia Wheel/2(T_c_inertia)  "T_c_inertia"
  Magnetic coils/1(T_coils) -> Sum/2, To Workspace1/1
  Subtract/1 -> Magnetic coils/1(T_Control), Scope/2  "T_c_coils"
  Constant/1 -> Product/1
  b_measured/1 -> Magnetic coils/2(b_measured)
  w_measured/1 -> Inertia Wheel/1(w_measured)

== system spacecraft_attitude_model/Disturbances Torque/Air Drag ==
  note: ASSUZNIONI:
      | - Il raggio dal centro di massa del Satellite
      | al centro di pressione di ogni superficie
      | è considerato lo stesso che ho usato per l'SRP
      | - qua ho messo l'altezza a 600 km
  v_rB_versor : Inport
  A_Cross : Subsystem
  Divide : Product  Inputs=*/
  Norm : Subsystem
  Square : Math  Operator=square
  Subsystem1 : Subsystem
  Subsystem2 : Subsystem
  Sum : Sum  Inputs=|++++++++++
  To Workspace : ToWorkspace  VariableName=T_Drag  SampleTime=-1
      settings: Save2DSignal=2-D array (concatenate along first dimension)
  T_Drag : Outport
  wires:
  A_Cross/1(A_cross1) -> Subsystem1/3(A_cross1)  "A_cross1"
  A_Cross/2(A_cross2) -> Subsystem1/4(A_cross2)
  A_Cross/3(A_cross3) -> Subsystem1/5(A_cross3)
  A_Cross/4(A_cross4) -> Subsystem1/6(A_cross4)
  A_Cross/5(A_cross5) -> Subsystem1/7(A_cross5)
  A_Cross/6(A_cross6) -> Subsystem1/8(A_cross6)
  A_Cross/7(A_cross7) -> Subsystem1/9(A_cross7)
  A_Cross/8(A_cross8) -> Subsystem1/10(A_cross8)
  A_Cross/9(A_cross9) -> Subsystem1/11(A_cross9)
  A_Cross/10(A_cross10) -> Subsystem1/12(A_cross10)
  Subsystem2/1(M1) -> Sum/1
  Subsystem2/2(M2) -> Sum/2
  Subsystem2/3(M3) -> Sum/3
  Subsystem2/8(M8) -> Sum/8
  Subsystem2/5(M5) -> Sum/5
  Subsystem2/4(M4) -> Sum/4
  Subsystem2/7(M7) -> Sum/7
  Subsystem2/10(M10) -> Sum/10
  Subsystem2/9(M9) -> Sum/9
  Subsystem2/6(M6) -> Sum/6
  Subsystem1/1(f1) -> Subsystem2/1(b1)
  Subsystem1/2(f2) -> Subsystem2/2(b2)
  Subsystem1/3(f3) -> Subsystem2/3(b3)
  Subsystem1/4(f4) -> Subsystem2/4(b4)
  Subsystem1/5(f5) -> Subsystem2/5(b5)
  Subsystem1/6(f6) -> Subsystem2/6(b6)
  Subsystem1/7(f7) -> Subsystem2/7(b7)
  Subsystem1/8(f8) -> Subsystem2/8(b8)
  Subsystem1/9(f9) -> Subsystem2/9(b9)
  Subsystem1/10(f10) -> Subsystem2/10(b10)
  Sum/1 -> To Workspace/1, T_Drag/1
  v_rB_versor/1 -> Norm/1(In1), Divide/1
  Norm/1(v_rB_norm) -> Divide/2, Square/1
  Divide/1 -> Subsystem1/2(v_rB_versor), A_Cross/1(v_rB_versor)
  Square/1 -> Subsystem1/1(v_rB^2)

== system spacecraft_attitude_model/Disturbances Torque/Gravity Gradient ==
  A_BL : Inport
  w : Inport  Port=2
  Gravity Gradient : Subsystem
  Scope : Scope
  To Workspace : ToWorkspace  VariableName=T_GG  SampleTime=-1
      settings: Save2DSignal=2-D array (concatenate along first dimension)
  w_dot to torque : Subsystem
  w_dot_GG : Outport
  "T_GG " : Outport  Port=2
  wires:
  w_dot to torque/1(T_GG) -> "T_GG "/1, Scope/1, To Workspace/1
  w/1 -> w_dot to torque/1(w)
  A_BL/1 -> Gravity Gradient/1(A_BL)
  Gravity Gradient/1(w_dot_GG) -> w_dot to torque/2(w_dot_GG), w_dot_GG/1

== system spacecraft_attitude_model/Disturbances Torque/Magnetic_Torque ==
  b_B : Inport
  Constant : Constant  Value=j_B
  Cross Product : matrix_library/Cross Product
  Scope : Scope
  To Workspace : ToWorkspace  VariableName=T_M  SampleTime=-1
      settings: Save2DSignal=2-D array (concatenate along first dimension)
  T_B : Outport
  wires:
  Constant/1 -> Cross Product/1
  b_B/1 -> Cross Product/2
  Cross Product/1 -> To Workspace/1, Scope/1, T_B/1

== system spacecraft_attitude_model/Disturbances Torque/Solar_Radiation_Torque ==
  S_B : Inport
  Divide1 : Product  Inputs=*/
  Norm : Subsystem
  SQR Force body 10 : Subsystem
  SQR Force body 6 : Subsystem
  SQR Force body 7 : Subsystem
  SQR Force body 8 : Subsystem
  SQR Force body 9 : Subsystem
  SQR Torque body 4 : Subsystem
  SQR Torque body 5 : Subsystem
  SQR torque body 1 : Subsystem
  SQR torque body 3 : Subsystem
  SQR torquw body 2 : Subsystem
  Scope : Scope
  Sum : Sum  Inputs=++++++++++
  To Workspace2 : ToWorkspace  VariableName=T_sun_tot  SampleTime=-1
      settings: Save2DSignal=2-D array (concatenate along first dimension)
  T sun : Outport
  wires:
  SQR Force body 6/1(T6) -> Sum/6
  SQR Force body 9/1(T9) -> Sum/9
  SQR torquw body 2/1(T2) -> Sum/2
  SQR Force body 10/1(T10) -> Sum/10
  SQR torque body 3/1(T3) -> Sum/3
  SQR torque body 1/1(T1) -> Sum/1
  SQR Force body 7/1(T7) -> Sum/7
  SQR Torque body 4/1(T4) -> Sum/4
  SQR Torque body 5/1(T5) -> Sum/5
  Sum/1 -> To Workspace2/1, Scope/1, T sun/1
  SQR Force body 8/1(T8) -> Sum/8
  Divide1/1 -> SQR Torque body 5/1(norm S_B), SQR Force body 6/1(norm S_B), SQR Force body 7/1(norm S_B), SQR Force body 8/1(norm S_B), SQR Force body 10/1(norm S_B), SQR Force body 9/1(norm S_B), SQR Torque body 4/1(norm S_B), SQR torque body 3/1(norm S_B), SQR torquw body 2/1(norm S_B), SQR torque body 1/1(norm S_B)
  Norm/1(Out1) -> Divide1/2  "r_norm"
  S_B/1 -> Divide1/1, Norm/1(In1)

== system spacecraft_attitude_model/Disturbances Torque/torque to w_dot_B ==
  T_B : Inport
  Constant1 : Constant  Value=J
  Divide : Product  Inputs=*/  Multiplication=Matrix(*)
  w_dot_B : Outport
  wires:
  Divide/1 -> w_dot_B/1
  T_B/1 -> Divide/1
  Constant1/1 -> Divide/2

== system spacecraft_attitude_model/Disturbances Torque/torque to w_dot_Drag ==
  T_Drag : Inport
  Constant1 : Constant  Value=J
  Divide : Product  Inputs=*/  Multiplication=Matrix(*)
  w_dot_Drag : Outport
  wires:
  Divide/1 -> w_dot_Drag/1
  T_Drag/1 -> Divide/1
  Constant1/1 -> Divide/2

== system spacecraft_attitude_model/Disturbances Torque/torque to w_dot_SRP ==
  T_S : Inport
  Constant1 : Constant  Value=J
  Divide : Product  Inputs=*/  Multiplication=Matrix(*)
  "w_dot_SRP " : Outport
  wires:
  Divide/1 -> "w_dot_SRP "/1
  T_S/1 -> Divide/1
  Constant1/1 -> Divide/2

== system spacecraft_attitude_model/Envoirment/Model ==
  r_N : Inport
  Magnetic Field : Subsystem
  Sun_Direction : Subsystem
  b_N : Outport
  S_N : Outport  Port=2
  wires:
  Sun_Direction/1(S_N) -> S_N/1
  r_N/1 -> Magnetic Field/1(r_N)
  Magnetic Field/1(b_N) -> b_N/1

== system spacecraft_attitude_model/Envoirment/Two_Body_Keplerian_Dynamics ==
  2BP : Subsystem
  Subsystem : Subsystem
  r_N : Outport
  Theta : Outport  Port=2
  wires:
  2BP/1(Theta) -> Theta/1, Subsystem/1(Theta)
  Subsystem/1(r_N) -> r_N/1

== system spacecraft_attitude_model/Inetial_to_Body/v_rel ==
  r_N : Inport
  Constant1 : Constant  Value=v0'
  Cross Product : matrix_library/Cross Product
  Sum : Sum  Inputs=|+-
  Transpose : Math  Operator=transpose
  Transpose1 : Math  Operator=transpose
  wE : Constant  Value=[0;0;w_E]
  v_rN : Outport
  wires:
  wE/1 -> Transpose1/1
  Constant1/1 -> Sum/1
  Sum/1 -> v_rN/1
  Cross Product/1 -> Sum/2
  r_N/1 -> Transpose/1
  Transpose/1 -> Cross Product/2
  Transpose1/1 -> Cross Product/1

== system spacecraft_attitude_model/Kinematics/quaternions ==
  w : Inport
  Divide1 : Product  Inputs=*/
  Gain : Gain  Gain=1/2
  Integrator : Integrator  InitialCondition=q0
  Matrix Multiply : Product  Multiplication=Matrix(*)
  Norm : Subsystem
  Omega(t) : Subsystem
  Scope : Scope
  To Workspace : ToWorkspace  VariableName=q  SampleTime=-1
  q : Outport
  wires:
  Omega(t)/1(Out1) -> Matrix Multiply/1
  w/1 -> Omega(t)/1(In1)
  Matrix Multiply/1 -> Gain/1
  Gain/1 -> Integrator/1
  Integrator/1 -> Divide1/1, Norm/1(In1)
  Norm/1(Out1) -> Divide1/2
  Divide1/1 -> Scope/1, q/1, To Workspace/1, Matrix Multiply/2
